simulink model "PM_fnc17_DevHarness_rate_limiter_r04"  (R2022a)
settings: Solver=FixedStepAuto  StartTime=0.0  StopTime=60  FixedStep=fixedsteprate_s  RelTol=1e-3
values from neighbouring files (symbols this model uses):
  fixedsteprate_s = rate_s    (= 0.01)    [PM_fnc1000_tc01_iter01_testsignal_builder.m]    (also in PM_fnc21_tc01_iter01_testsignal_builder.m; PM_fnc22_tc01_iter01_testsignal_builder.m)
libraries: PM_lib x1
settings Model: NumberOfSteps=2  Creator=306427  LastModifiedBy=306427

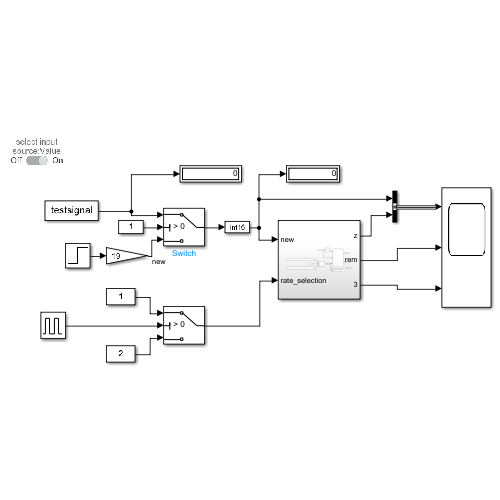
[thumbnail: Simulink's stored preview of the top-level diagram]
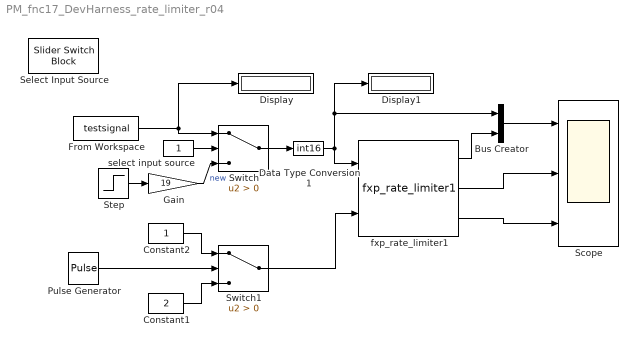
== system PM_fnc17_DevHarness_rate_limiter_r04 ==
  Bus Creator : BusCreator  Inputs=2
  Constant1 : Constant  Value=2
  Constant2 : Constant
  Data Type Conversion1 : DataTypeConversion  OutDataTypeStr=int16  SaturateOnIntegerOverflow=off  RndMeth=Floor
  Display : Display
  Display1 : Display
  From Workspace : FromWorkspace  VariableName=testsignal  SampleTime=fixedsteprate_s
  Gain : Gain  Gain=19  OutDataTypeStr=int16  ParamDataTypeStr=Inherit: Same as input
  Pulse Generator : DiscretePulseGenerator  PulseType=Time based  Period=50  PulseWidth=50
  Scope : Scope  NumInputPorts=3
  Select Input Source : SliderSwitchBlock
      settings: Values={{'Off', 'On'}, [0 1]}
  Step : Step  SampleTime=fixedsteprate_s
  Switch : Switch  Criteria=u2 > Threshold  SaturateOnIntegerOverflow=off  InputSameDT=off
  Switch1 : Switch  Criteria=u2 > Threshold  SaturateOnIntegerOverflow=off  InputSameDT=off
  fxp_rate_limiter1 : PM_lib/fxp_rate_limiter1  SystemSampleTime=-1  VariantActivationTime=update diagram  Latency=0  AutoFrameSizeCalculation=off
  select input source : Constant
  wires:
  Gain/1 -> Switch/3  "new"
  Bus Creator/1 -> Scope/1
  fxp_rate_limiter1/1 -> Bus Creator/2
  fxp_rate_limiter1/2 -> Scope/2
  select input source/1 -> Switch/2
  From Workspace/1 -> Display/1, Switch/1
  Switch/1 -> Data Type Conversion1/1
  Data Type Conversion1/1 -> fxp_rate_limiter1/1, Bus Creator/1, Display1/1
  Step/1 -> Gain/1
  Pulse Generator/1 -> Switch1/2
  Constant1/1 -> Switch1/3
  Constant2/1 -> Switch1/1
  Switch1/1 -> fxp_rate_limiter1/2
  fxp_rate_limiter1/3 -> Scope/3
